simulink model "ProjectileModel"  (R2020b)
settings: Solver=FixedStepAuto  StartTime=0.0  StopTime=6  FixedStep=1e-3  RelTol=1e-3
values from neighbouring files (symbols this model uses):
  D = 0.5*C*rho*A    (= 0.00128880775561)    [ProjectileModelParameter.m]
  g = 9.81    [ProjectileModelParameter.m]    (also in Variables.mat)
  m = 0.145    [ProjectileModelParameter.m]    (also in Variables.mat = 0.62)
  theta = 60    [ProjectileModelParameter.m]
  vx = v0*cosd(theta)    [ProjectileModelParameter.m]
  vy = v0*sind(theta)    [ProjectileModelParameter.m]
  x0 = -35    [ProjectileModelParameter.m]
  y0 = 0    [ProjectileModelParameter.m]
libraries: vrlib x7
settings Model: Creator=user  LastModifiedBy=user

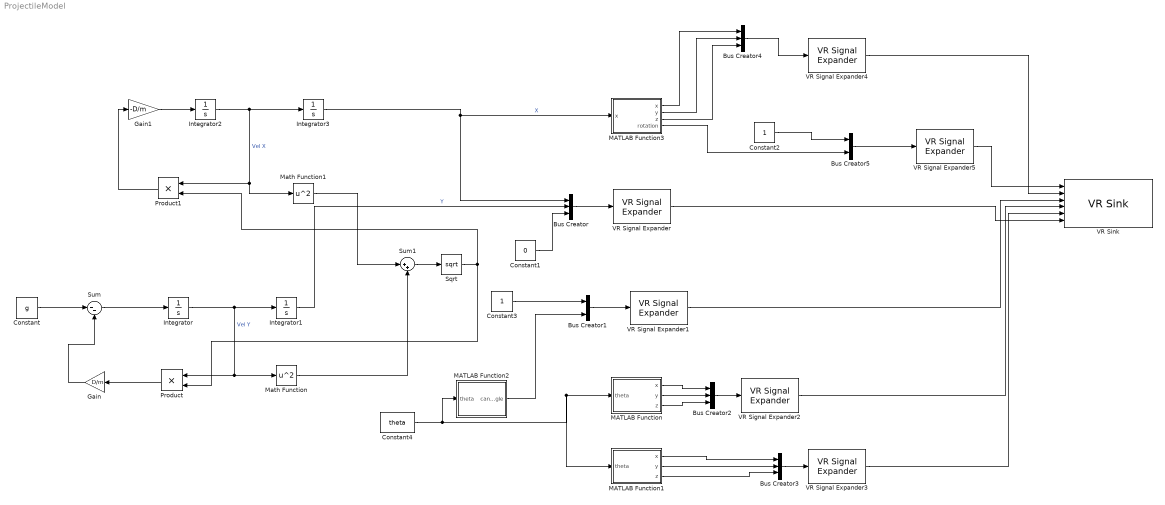
== system ProjectileModel ==
  Bus Creator{,2..4} (4 alike) : BusCreator  Inputs=3
  Bus Creator1 : BusCreator  Inputs=2
  Bus Creator5 : BusCreator  Inputs=2
  Constant : Constant  Value=g
  Constant1 : Constant  Value=0
  Constant2 : Constant
  Constant3 : Constant
  Constant4 : Constant  Value=theta
  Gain : Gain  Gain=D/m
  Gain1 : Gain  Gain=-D/m
  Integrator : Integrator  InitialCondition=vy  UpperSaturationLimit=1000  LowerSaturationLimit=0
  Integrator1 : Integrator  InitialCondition=y0
  Integrator2 : Integrator  InitialCondition=vx  UpperSaturationLimit=1000  LowerSaturationLimit=0
  Integrator3 : Integrator  InitialCondition=x0
  MATLAB Function : MATLAB Function  TreatAsAtomicUnit=on
  MATLAB Function1 : MATLAB Function  TreatAsAtomicUnit=on
  MATLAB Function2 : MATLAB Function  TreatAsAtomicUnit=on
  MATLAB Function3 : MATLAB Function  TreatAsAtomicUnit=on
  Math Function : Math  Operator=square  SaturateOnIntegerOverflow=on
  Math Function1 : Math  Operator=square  SaturateOnIntegerOverflow=on
  Product : Product
  Product1 : Product
  Sqrt : Sqrt  SaturateOnIntegerOverflow=on
  Sum : Sum  Inputs=|--
  Sum1 : Sum  Inputs=|++
  VR Signal Expander{,2..4} (4 alike) : vrlib/VR Signal Expander  outwidth=3  outidx=[1 2 3]
  VR Signal Expander1 : vrlib/VR Signal Expander  outwidth=4  outidx=[3 4]
  VR Signal Expander5 : vrlib/VR Signal Expander  outwidth=4  outidx=[3 4]
  VR Sink : vrlib/VR Sink  InstantiateOnLoad=on  SampleTime=0.05  ViewEnable=on  RemoteChange=off  RemoteView=off  FieldsWritten=Target.rotation.4.1.1.double#Target.translation.3.1.1.double#Cannon_body.rotation.4.1.1.double#Cannon_head_right.translation.3.1.1.double#Cannon_head_left.translation.3.1.1.double#Ball.translation.3.1.1.double  WorldFileName=BallMovement.wrl  AutoView=on  VideoDimensions=[]  AllowVariableSize=off
  wires:
  Constant/1 -> Sum/1
  Sum/1 -> Integrator/1
  Integrator/1 -> Product/1, Math Function/1, Integrator1/1  "Vel Y"
  Product/1 -> Gain/1
  Gain/1 -> Sum/2
  Math Function/1 -> Sum1/2
  Math Function1/1 -> Sum1/1
  Product1/1 -> Gain1/1
  Gain1/1 -> Integrator2/1
  Integrator2/1 -> Math Function1/1, Product1/1, Integrator3/1  "Vel X"
  Sum1/1 -> Sqrt/1
  Sqrt/1 -> Product/2, Product1/2
  Integrator3/1 -> MATLAB Function3/1("x "), Bus Creator/1  "X"
  Integrator1/1 -> Bus Creator/2  "Y"
  Constant1/1 -> Bus Creator/3
  Bus Creator/1 -> VR Signal Expander/1
  Bus Creator1/1 -> VR Signal Expander1/1
  Constant3/1 -> Bus Creator1/1
  Constant4/1 -> MATLAB Function2/1(theta), MATLAB Function1/1(theta), MATLAB Function/1(theta)
  MATLAB Function/1(x) -> Bus Creator2/1
  MATLAB Function/2(y) -> Bus Creator2/2
  MATLAB Function/3(z) -> Bus Creator2/3
  Bus Creator2/1 -> VR Signal Expander2/1
  MATLAB Function1/3(z) -> Bus Creator3/3
  Bus Creator3/1 -> VR Signal Expander3/1
  MATLAB Function1/1(x) -> Bus Creator3/1
  MATLAB Function1/2(y) -> Bus Creator3/2
  MATLAB Function2/1(can_angle) -> Bus Creator1/2
  VR Signal Expander1/1 -> VR Sink/3
  VR Signal Expander2/1 -> VR Sink/4
  VR Signal Expander3/1 -> VR Sink/5
  VR Signal Expander/1 -> VR Sink/6
  MATLAB Function3/2(y) -> Bus Creator4/2
  MATLAB Function3/4(rotation) -> Bus Creator5/2
  MATLAB Function3/1(x) -> Bus Creator4/1
  MATLAB Function3/3(z) -> Bus Creator4/3
  Bus Creator4/1 -> VR Signal Expander4/1
  Constant2/1 -> Bus Creator5/1
  Bus Creator5/1 -> VR Signal Expander5/1
  VR Signal Expander5/1 -> VR Sink/1
  VR Signal Expander4/1 -> VR Sink/2

== matlab function ProjectileModel/MATLAB Function1 ==
  data: x output; theta input; y output; z output
function [x,y,z] = fcn(theta)
if theta<=80 && theta>70
    x=-29.2;
elseif theta<=70 && theta>60
    x=-30.2;
elseif theta<=60
    x=-31.2;
else
    x=-28.2;
end
y = -4.1040;
z=15;
end

== matlab function ProjectileModel/MATLAB Function ==
  data: x output; theta input; y output; z output
function [x,y,z] = fcn(theta)
if theta<=80 && theta>70
    x=-27.2;
elseif theta<=70 && theta>60
    x=-28.2;
elseif theta<=60
    x=-29.2;
else
    x=-26.2;
end
y = -4.1040;
z=25.0000;
end

== matlab function ProjectileModel/MATLAB Function2 ==
  data: can_angle output; theta input
function can_angle= fcn(theta)
if theta<=85 && theta>75
    can_angle=-10;
elseif theta<=75 && theta>65
    can_angle=-70;
elseif theta<=65 && theta>55
    can_angle=40;
elseif theta<=55 && theta>=45
    can_angle=-45;
elseif theta<45
    can_angle=-80;
else
    can_angle=0;
end
end

== matlab function ProjectileModel/MATLAB Function3 ==
  data: x output; x input; y output; z output; rotation output
function [x,y,z,rotation] = fcn(x)
 if x>=34
     y=-3;
     rotation=-90;
 else
     y=3;
     rotation=0;
 end
 x=35;
 z=0;
end
